simulink model "Solar"  (R2019a)
settings: Solver=ode45  StartTime=0.0  StopTime=10.0  RelTol=1e-3  EnableMultiTasking=on
settings Model: Creator=student  LastModifiedBy=OWNER
settings DataIOCC: LimitDataPoints=on  SaveFormat=Array  SignalLoggingSaveFormat=ModelDataLogs  ReturnWorkspaceOutputs=off
settings OptimizationCC: ExpressionDepthLimit=2147483647  InitFltsAndDblsToZero=on  LifeSpan=inf
settings DebuggingCC: SaveWithParameterizedLinksMsg=none  UnderspecifiedInitializationDetection=Classic  MergeDetectMultiDrivingBlocksExec=none  SolverPrmCheckMsg=warning  FcnCallInpInsideContextMsg=warning  StateNameClashWarn=warning  SFUnexpectedBacktrackingDiag=warning  SFNoUnconditionalDefaultTransitionDiag=warning  SFExecutionAtInitializationDiag=none  ArithmeticOperatorsInVariantConditions=warning
settings HardwareCC: ProdBitPerPointer=32  ProdBitPerSizeT=32  ProdBitPerPtrDiffT=32  ProdLargestAtomicFloat=None  ProdIntDivRoundTo=Undefined  ProdEndianess=Unspecified  ProdWordSize=32  ProdHWDeviceType=32-bit Generic
settings ModelReferenceCC: PropagateSignalLabelsOutOfModel=off
settings SFSimCC: SimUseLocalCustomCode=off
settings RTWCC: RTWUseLocalCustomCode=off
settings CodeAppCC: StateflowObjectComments=on
settings GRTTargetCC: TargetFcnLib=ansi_tfl_tmw.mat  TargetLangStandard=C89/C90 (ANSI)  GeneratePreprocessorConditionals=Disable all  CombineOutputUpdateFcns=off  GRTInterface=on
settings ConfigComp: CovMetricSettings=dw  CovHtmlReporting=on  CovSaveCumulativeToWorkspaceVar=on  CovSaveSingleToWorkspaceVar=on  CovExternalEMLEnable=off

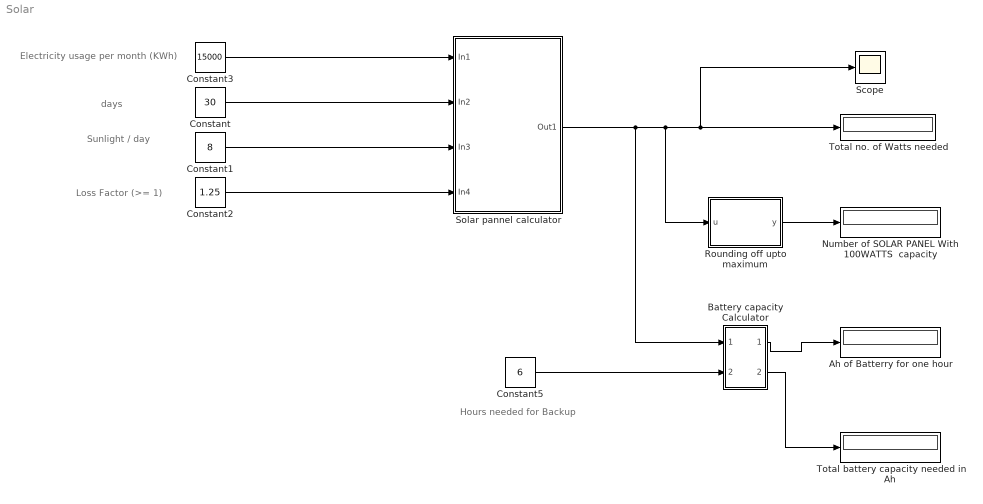
== system Solar ==
  note: Electricity usage per month (KWh)
  note: days
  note: Sunlight / day
  note: Loss Factor (>= 1)
  note: Hours needed for Backup
  Ah of Batterry for one hour : Display
  Battery capacity Calculator : Subsystem
  Constant : Constant  Value=30
  Constant1 : Constant  Value=8
  Constant2 : Constant  Value=1.25
  Constant3 : Constant  Value=15000
  Constant5 : Constant  Value=6
  Number of SOLAR PANEL With 100WATTS  capacity : Display
  Rounding off upto maximum : MATLAB Function  TreatAsAtomicUnit=on
  Scope : Scope
  Solar pannel calculator : Subsystem
  Total battery capacity needed in Ah : Display
  "Total no. of Watts needed " : Display
  wires:
  Constant3/1 -> Solar pannel calculator/1(In1)
  Constant/1 -> Solar pannel calculator/2(In2)
  Constant1/1 -> Solar pannel calculator/3(In3)
  Constant2/1 -> Solar pannel calculator/4(In4)
  Solar pannel calculator/1(Out1) -> Battery capacity Calculator/1(In1), Scope/1, "Total no. of Watts needed "/1, Rounding off upto maximum/1(u)
  Constant5/1 -> Battery capacity Calculator/2(In2)
  Battery capacity Calculator/2(Out2) -> Total battery capacity needed in Ah/1
  Rounding off upto maximum/1(y) -> Number of SOLAR PANEL With 100WATTS  capacity/1
  Battery capacity Calculator/1(Out1) -> Ah of Batterry for one hour/1

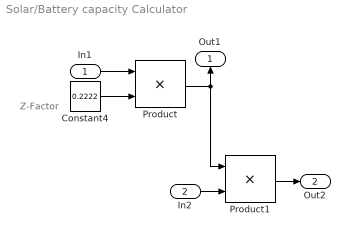
== system Solar/Battery capacity Calculator ==
  note: Z-Factor
  In1 : Inport
  In2 : Inport  Port=2
  Constant4 : Constant  Value=0.2222
  Product : Product  RndMeth=Zero
  Product1 : Product  RndMeth=Zero
  Out1 : Outport
  Out2 : Outport  Port=2
  wires:
  Constant4/1 -> Product/2
  Product/1 -> Product1/1, Out1/1
  In1/1 -> Product/1
  Product1/1 -> Out2/1
  In2/1 -> Product1/2

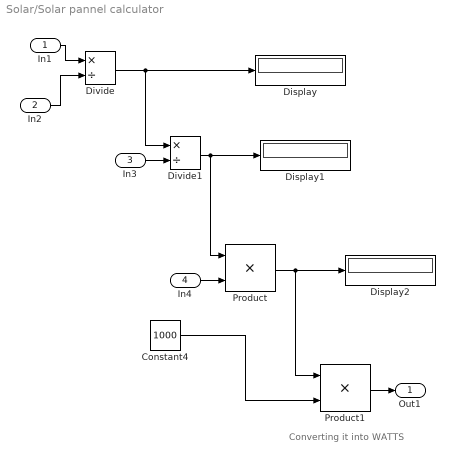
== system Solar/Solar pannel calculator ==
  note: Converting it into WATTS
  In1 : Inport
  In2 : Inport  Port=2
  In3 : Inport  Port=3
  In4 : Inport  Port=4
  Constant4 : Constant  Value=1000
  Display : Display
  Display1 : Display
  Display2 : Display
  Divide : Product  Inputs=*/
  Divide1 : Product  Inputs=*/
  Product : Product  RndMeth=Zero
  Product1 : Product  RndMeth=Zero
  Out1 : Outport
  wires:
  Divide/1 -> Display/1, Divide1/1
  Divide1/1 -> Display1/1, Product/1
  Product/1 -> Display2/1, Product1/1
  Constant4/1 -> Product1/2
  In1/1 -> Divide/1
  In2/1 -> Divide/2
  In3/1 -> Divide1/2
  In4/1 -> Product/2
  Product1/1 -> Out1/1

== matlab function Solar/Rounding off upto maximum ==
  data: u input; y output
function y = fcn(u)
% This block supports an embeddable subset of the MATLAB language.
% See the help menu for details. 
y = floor(u / 100)+1;
